simulink model "simulation"  (R2018a)
settings: Solver=VariableStepAuto  StartTime=0.0  StopTime=40  RelTol=1e-3
values from neighbouring files (symbols this model uses):
  A = [0 1 0; 0 0 1; 0 0 0]    [Q_learning.m]
  B = [0; 0; 1]    [Q_learning.m]
undefined symbols (not defined in the file or in its folder): Kest, x
settings Model: Creator=harry  LastModifiedBy=harry

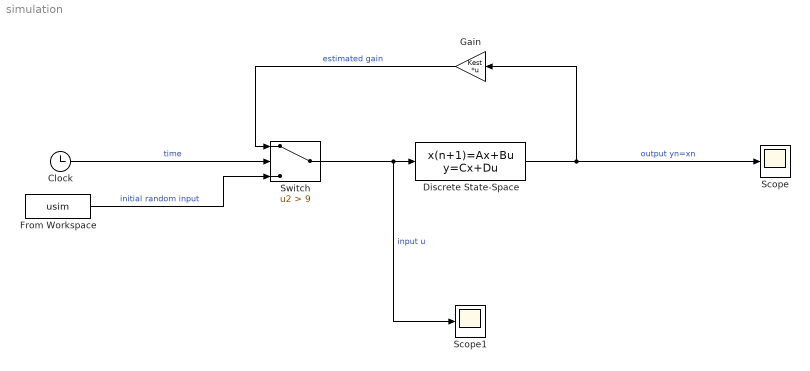
== system simulation ==
  Clock : Clock
  Discrete State-Space : DiscreteStateSpace  A=A  B=B  C=eye(3)  D=[0; 0; 0]  InitialCondition=x(:,1)  SampleTime=-1
  From Workspace : FromWorkspace  VariableName=usim  SampleTime=0
  Gain : Gain  Gain=Kest  Multiplication=Matrix(K*u)
  Scope : Scope
  Scope1 : Scope
  Switch : Switch  Criteria=u2 > Threshold  Threshold=9
  wires:
  Discrete State-Space/1 -> Gain/1, Scope/1  "output yn=xn"
  Switch/1 -> Scope1/1, Discrete State-Space/1  "input u"
  Clock/1 -> Switch/2  "time"
  From Workspace/1 -> Switch/3  "initial random input"
  Gain/1 -> Switch/1  "estimated gain"
